simulink model "vertical_smm_3d_with_xz_lqr"  (R2015a)
settings: Solver=FixedStepDiscrete  SolverMode=SingleTasking  StartTime=0.0  StopTime=inf  FixedStep=sample_time  RelTol=1e-3
values from neighbouring files (symbols this model uses):
  forward_dx_of_dxstar = [-1.33773437568 -1.28773437515 -1.23773437461 -1.18773437408 -1.13773437355 -1.08773437301 -1.03773437248 -0.987734371946 -0.937734371413 -0.887734370879 -0.837734370532 -0.787734370254 ... (27552 elements, 41x21x32)]    [ref_trajs.mat]
  forward_x_of_dxstar = [0.243075305346 0.235858801492 0.228642297639 0.221425793786 0.214209289933 0.206992786079 0.199776282226 0.192559778373 0.18534327452 0.178126770666 0.17091026684 0.163693763058 ... (27552 elements, 41x21x32)]    [ref_trajs.mat]
  target_dx_range = [-1 -0.95 -0.9 -0.85 -0.8 -0.75 -0.7 -0.65 -0.6 -0.55 -0.5 -0.45 ... (41 elements, 1x41)]    [ref_trajs.mat]
undefined symbols (not defined in the file or in its folder): A1_notch_f1, A2_notch_f1, A_kalman_fourbar_gear, A_kalman_swing_load, A_kalman_transverse, A_kalman_vertical, A_lpf_accelerometer, A_lpf_dtau, A_lpf_fourbar_angles, A_lpf_imu, A_lpf_lateral_angle, B1_lpf_accelerometer, B1_lpf_dtau, B1_lpf_fourbar_angles, B1_lpf_imu, B1_lpf_lateral_angle, B1_notch_f1, B2_lpf_accelerometer, B2_lpf_dtau, B2_lpf_fourbar_angles, B2_lpf_imu, B2_lpf_lateral_angle, B2_notch_f1, B_dx_versus_x0, B_kalman_fourbar_gear, B_kalman_swing_load, B_kalman_transverse, B_kalman_vertical, backwards_K_sag_of_t, backwards_P_sag_of_t, C_kalman_fourbar_gear, C_kalman_swing_load, C_kalman_transverse, C_kalman_vertical, com_leg_motor, com_torso, contact_threshold, control_start_time, d_ankle_to_foot, d_vertical_com, desired_com_forward_velocity, desired_com_lateral_velocity, desired_initial_leg_roll_left, desired_initial_leg_roll_right, desired_stance_beta2, desired_standing_torso_pitch, desired_standing_torso_roll, desired_standing_z, desired_torso_pitch, desired_torso_roll, Discrete, enable_bouncing, fcut_contact, fdesignblkfcn, g, gcbh, HIP_MTR_MAX_CONT_TORQUE, HIP_MTR_MAX_TORQUE, i_leg_motor, i_robot ... (+91)
libraries: simulink x33, ctrlSharedLib x11, dsparch4 x10, dspfdesign x2
(part 1 of 7)
settings Model: CovSFcnEnable=off  Creator=wmartin  LastModifiedBy=wmartin
settings SolverCC: EnableConcurrentExecution=on
settings DataIOCC: LimitDataPoints=off  MaxDataPoints=1000000000  SaveFormat=StructureWithTime  SignalLogging=off  DSMLogging=off  VisualizeSimOutput=off
settings OptimizationCC: BlockReduction=off  OptimizeBlockIOStorage=off  BufferReuse=off  GlobalBufferReuse=off  ExpressionFolding=off  ExpressionDepthLimit=2147483647  LocalBlockOutputs=off  SimCompilerOptimization=on
settings DebuggingCC: UnderspecifiedInitializationDetection=Classic  MergeDetectMultiDrivingBlocksExec=none  SolverPrmCheckMsg=warning  StateNameClashWarn=warning
settings HardwareCC: ProdIntDivRoundTo=Zero  ProdEndianess=LittleEndian  ProdLongLongMode=on  ProdHWDeviceType=Generic->32-bit x86 compatible
settings ModelReferenceCC: UpdateModelReferenceTargets=IfOutOfDate  ModelReferenceNumInstancesAllowed=Single  ModelReferenceMinAlgLoopOccurrences=on
settings RTWCC: SystemTargetFile=slrt.tlc  TemplateMakefile=slrt_default_tmf  Description=Simulink Real-Time  RTWVerbose=off  RTWCompilerOptimization=on
settings CodeAppCC: MaxIdLength=256
settings SimulinkRealTimeCC: GeneratePreprocessorConditionals=Disable all  RL32LogBufSizeModifier=1e8

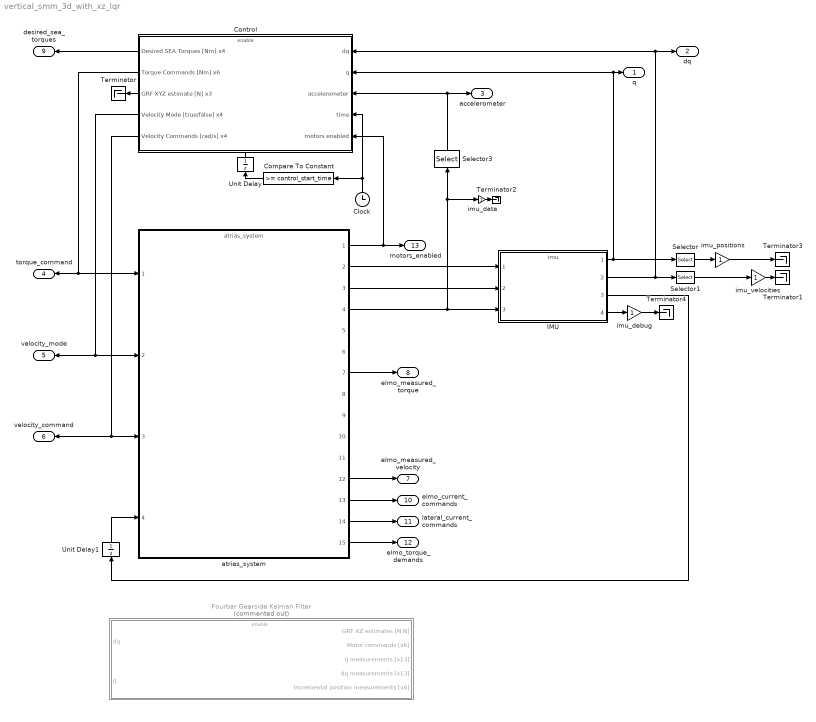
== system vertical_smm_3d_with_xz_lqr ==
  Clock : Clock
  Compare To Constant : simulink/Logic and Bit Operations/Compare To Constant  relop=>=  const=control_start_time  OutDataTypeStr=boolean
  Control : Subsystem
  Fourbar Gearside Kalman Filter : Subsystem  Commented=on
  IMU : ModelReference  ModelNameDialog=imu  SimulationMode=Normal  ModelReferenceVersion=1.2455  CopyOfModelName=imu  DefaultDataLogging=on
  Selector : Selector  InputPortWidth=13  Indices=[11 12 13]
  Selector1 : Selector  InputPortWidth=13  Indices=[11 12 13]
  Selector3 : Selector  InputPortWidth=9  Indices=[4 5 6]
  Terminator{,1..4} (5 alike) : Terminator
  Unit Delay : UnitDelay  SampleTime=-1
  Unit Delay1 : UnitDelay  SampleTime=-1
  atrias_system : ModelReference  ModelNameDialog=atrias_system  SimulationMode=Normal  ModelReferenceVersion=1.2965  CopyOfModelName=atrias_system  DefaultDataLogging=on
  imu_data : Gain
  imu_debug : Gain
  imu_positions : Gain
  imu_velocities : Gain
  q : Outport  SampleTime=sample_time
  dq : Outport  Port=2  SampleTime=sample_time
  accelerometer : Outport  Port=3  SampleTime=sample_time
  torque_command : Outport  Port=4  SampleTime=sample_time
  velocity_mode : Outport  Port=5  SampleTime=sample_time
  velocity_command : Outport  Port=6  SampleTime=sample_time
  elmo_measured_velocity : Outport  Port=7  SampleTime=sample_time
  elmo_measured_torque : Outport  Port=8  SampleTime=sample_time
  desired_sea_torques : Outport  Port=9  SampleTime=sample_time
  elmo_current_commands : Outport  Port=10  SampleTime=sample_time
  lateral_current_commands : Outport  Port=11  SampleTime=sample_time
  elmo_torque_demands : Outport  Port=12  SampleTime=sample_time
  motors_enabled : Outport  Port=13  SampleTime=sample_time
  wires:
  Compare To Constant/1 -> Unit Delay/1
  imu_data/1 -> Terminator2/1
  imu_velocities/1 -> Terminator1/1
  imu_positions/1 -> Terminator3/1
  imu_debug/1 -> Terminator4/1
  IMU/4 -> imu_debug/1
  Selector/1 -> imu_positions/1
  Selector1/1 -> imu_velocities/1
  atrias_system/2 -> IMU/1
  IMU/1 -> Selector/1, Control/2(q), q/1
  Control/2(Torque Commands [Nm] x6) -> atrias_system/1, torque_command/1
  atrias_system/3 -> IMU/2
  atrias_system/4 -> Selector3/1, imu_data/1, IMU/3
  IMU/3 -> Unit Delay1/1
  Unit Delay/1 -> Control/Enable
  IMU/2 -> Selector1/1, Control/1(dq), dq/1
  Control/5(Velocity Commands [rad/s] x4) -> velocity_command/1, atrias_system/3
  Control/4(Velocity Mode [true/false] x4) -> velocity_mode/1, atrias_system/2
  Selector3/1 -> Control/3(accelerometer), accelerometer/1
  Control/1(Desired SEA Torques [Nm] x4) -> desired_sea_torques/1
  Clock/1 -> Control/4(time), Compare To Constant/1
  Control/3(GRF XYZ estimate [N] x3) -> Terminator/1
  atrias_system/15 -> elmo_torque_demands/1
  atrias_system/14 -> lateral_current_commands/1
  atrias_system/13 -> elmo_current_commands/1
  atrias_system/12 -> elmo_measured_velocity/1
  atrias_system/7 -> elmo_measured_torque/1
  atrias_system/1 -> Control/5(motors enabled), motors_enabled/1
  Unit Delay1/1 -> atrias_system/4

== system vertical_smm_3d_with_xz_lqr/Control ==
  dq : Inport
  q : Inport  Port=2
  accelerometer : Inport  Port=3
  time : Inport  Port=4
  motors enabled : Inport  Port=5
  Enable : EnablePort  StatesWhenEnabling=reset  PropagateVarSize=During execution  ShowOutputPort=on
  Actuator Control : ModelReference  ModelNameDialog=actuator_control  SimulationMode=Normal  ModelReferenceVersion=1.1249  CopyOfModelName=actuator_control  DefaultDataLogging=on
  Actuator Control with Torque SEA commands : Subsystem  Commented=on
  Behavior Control : Subsystem
  Compute Body Frame Accelerations : Subsystem
  Detect Change : simulink/Logic and Bit Operations/Detect Change  vinit=0  InputProcessing=Inherited  OutDataTypeStr=boolean
  Filter Velocities : Subsystem
  Mux : Mux
  Desired SEA Torques [Nm] x4 : Outport  InitialOutput=[0 0 0 0]
  Torque Commands [Nm] x6 : Outport  Port=2  InitialOutput=[0 0 0 0 0 0]
  GRF XYZ estimate [N] x3 : Outport  Port=3  InitialOutput=[0 0 0]
  Velocity Mode [true/false] x4 : Outport  Port=4  InitialOutput=[false false false false]
  Velocity Commands [rad/s] x4 : Outport  Port=5  InitialOutput=[0 0 0 0]
  wires:
  Behavior Control/1(Torque Commands [Nm] x6) -> Actuator Control/2
  Behavior Control/2(Velocity Commands [rad/s] x4) -> Actuator Control/3
  Behavior Control/3(Stance / Swing Control [1/0] x4) -> Actuator Control/4
  time/1 -> Actuator Control/5, Behavior Control/5(time)
  Detect Change/1 -> Mux/1, Mux/2, Mux/3, Mux/4
  motors enabled/1 -> Detect Change/1
  Mux/1 -> Actuator Control/1
  Actuator Control/4 -> Desired SEA Torques [Nm] x4/1
  Enable/1 -> Behavior Control/1(Enabled [true/false])
  Compute Body Frame Accelerations/1(accelerations [m/s^2] x3) -> Behavior Control/2(Body XYZ Acceleration [m/s^2] x3)
  accelerometer/1 -> Compute Body Frame Accelerations/1(accelerometer [g] x3)
  Actuator Control/3 -> Velocity Commands [rad/s] x4/1
  Actuator Control/2 -> Velocity Mode [true/false] x4/1
  dq/1 -> Actuator Control/7, Filter Velocities/1(raw dq)
  Filter Velocities/1(filtered dq) -> Behavior Control/3(dq)
  Behavior Control/4(GRF XYZ estimates [N N N]) -> GRF XYZ estimate [N] x3/1
  Actuator Control/1 -> Torque Commands [Nm] x6/1
  q/1 -> Actuator Control/6, Behavior Control/4(q)

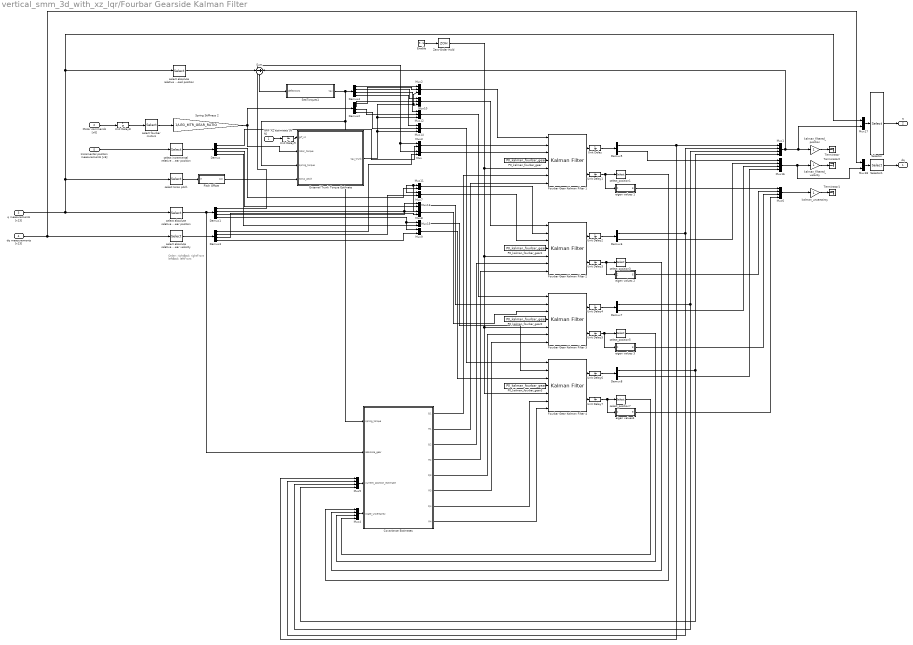
== system vertical_smm_3d_with_xz_lqr/Fourbar Gearside Kalman Filter ==
  note: Order:
      | rightBack
      | rightFront
      | leftBack
      | leftFront
  GRF XZ estimates [N N] : Inport  SampleTime=sample_time
  Motor commands [x6] : Inport  Port=2  SampleTime=sample_time
  q measurements [x13] : Inport  Port=3  SampleTime=sample_time
  dq measurements [x13] : Inport  Port=4  SampleTime=sample_time
  Incremental position measurements [x6] : Inport  Port=5  SampleTime=sample_time
  Enable : EnablePort  ShowOutputPort=on
  Covariance Estimates : MATLAB Function  TreatAsAtomicUnit=on
  Demux{,1..4} (5 alike) : Demux
  Demux{5..8} (4 alike) : Demux  Outputs=2
  External Trunk Torque Estimate : MATLAB Function  TreatAsAtomicUnit=on
  Fourbar Gear Kalman Filter {1..4} (4 alike) : ctrlSharedLib/Kalman Filter  TimeDomain=Discrete-Time  UseCurrentEstimator=on  ModelSource=Individual A, B, C, D matrices  ModelSourceVariable=A_kf  A=A_kalman_fourbar_gear  B=B_kalman_fourbar_gear  C=C_kalman_fourbar_gear  D=0  NumberOfStates=2  NumberOfInputs=1  NumberOfOutputs=2  InitialEstimateSource=Input port  X0=initial_dx_estimate  P0=P0_kalman_transverse  UseK=off  UseGH=on  NumberOfProcessNoiseInputs=1  G=G_kalman_fourbar_gear  TimeInvariantG=on  H=0  TimeInvariantH=on  Q=1  TimeInvariantQ=off  R=1  TimeInvariantR=off  N=0  TimeInvariantN=on  AddInputPort=on  AddEnablePort=off  ExternalReset=Either  OutputEstimatedY=off  OutputP=on  Ts=sample_time
  Mux{,3,7..9,11,13,15,17..18} (10 alike) : Mux  Inputs=2
  Mux{1,4..6,16} (5 alike) : Mux
  Mux{2,10,12,14} (4 alike) : Mux  Inputs=3
  P0_kalman_fourbar_gear{,1..3} (4 alike) : Constant  Value=P0_kalman_fourbar_gear
  Pitch Offset : Subsystem
  SeaTorques1 : MATLAB Function  TreatAsAtomicUnit=on
  Selector : Selector  InputPortWidth=17  Indices=[1 14 3 15 5 16 7 17 9 10 11 12 13]
  Selector1 : Selector  InputPortWidth=17  Indices=[1 14 3 15 5 16 7 17 9 10 11 12 13]
  Spring Stiffness 2 : Gain  Gain=1/LEG_MTR_GEAR_RATIO
  Sum : Sum  Inputs=-|+
  Terminator : Terminator
  Terminator1 : Terminator
  Terminator2 : Terminator
  Unit Delay{,1..9} (10 alike) : UnitDelay  SampleTime=-1
  Zero-Order Hold : ZeroOrderHold  SampleTime=sample_time
  eigen values 1 : MATLAB Function  TreatAsAtomicUnit=on
  eigen values 2 : MATLAB Function  TreatAsAtomicUnit=on
  eigen values 3 : MATLAB Function  TreatAsAtomicUnit=on
  "eigen values4 " : MATLAB Function  TreatAsAtomicUnit=on
  kalman_filtered_position : Gain
  kalman_filtered_velocity : Gain
  kalman_uncertainty : Gain
  select absolute relative gear position : Selector  InputPortWidth=13  Indices=[2 4 6 8]
  select absolute relative gear velocity : Selector  InputPortWidth=13  Indices=[2 4 6 8]
  select absolute relative load position : Selector  InputPortWidth=13  Indices=[2 4 6 8]
  select fourbar motors : Selector  InputPortWidth=6  Indices=[1 2 3 4]
  select incremental relative gear position : Selector  InputPortWidth=6  Indices=[1 2 3 4]
  select torso pitch : Selector  InputPortWidth=13  Indices=[13]
  select_position{1,3,5,7} (4 alike) : Selector  NumberOfDimensions=2  InputPortWidth=2  IndexOptions=Index vector (dialog),Index vector (dialog)  Indices=[1],[1]  OutputSizes=1,1
  dq : Outport
  q : Outport  Port=2
  wires:
  select incremental relative gear position/1 -> Demux/1
  q measurements [x13]/1 -> select absolute relative gear position/1, Mux17/1, select absolute relative load position/1, select torso pitch/1
  Incremental position measurements [x6]/1 -> select incremental relative gear position/1
  Motor commands [x6]/1 -> Unit Delay8/1
  select fourbar motors/1 -> Spring Stiffness 2/1
  P0_kalman_fourbar_gear/1 -> Fourbar Gear Kalman Filter 1/4
  Mux/1 -> Fourbar Gear Kalman Filter 1/3
  select absolute relative gear velocity/1 -> Demux3/1
  dq measurements [x13]/1 -> Mux18/1, select absolute relative gear velocity/1
  Demux3/1 -> Mux/2
  GRF XZ estimates [N N]/1 -> Unit Delay9/1
  SeaTorques1/1(tau) -> Demux4/1, External Trunk Torque Estimate/3(spring_torque), Covariance Estimates/1(spring_torque)
  Fourbar Gear Kalman Filter 1/1 -> Unit Delay/1
  Demux5/1 -> Mux1/1, Mux5/1
  Mux1/1 -> Sum/2, Mux17/2, kalman_filtered_position/1
  select absolute relative load position/1 -> Sum/1
  Sum/1 -> SeaTorques1/1(deflections)
  External Trunk Torque Estimate/1(tau_trunk) -> Mux2/3, Mux10/3, Mux12/3, Mux14/3
  Demux4/1 -> Mux2/1
  Demux2/1 -> Mux2/2
  Mux2/1 -> Fourbar Gear Kalman Filter 1/1
  Demux/1 -> Mux3/2
  Demux1/1 -> Mux3/1, Mux/1
  Mux3/1 -> Fourbar Gear Kalman Filter 1/2
  Fourbar Gear Kalman Filter 1/2 -> Unit Delay1/1
  Mux4/1 -> Covariance Estimates/4(state_uncertainty)
  select absolute relative gear position/1 -> Covariance Estimates/2(absolute_gear), Demux1/1
  Mux5/1 -> Covariance Estimates/3(current_position_estimate)
  Covariance Estimates/1(Q1) -> Fourbar Gear Kalman Filter 1/6
  Covariance Estimates/2(R1) -> Fourbar Gear Kalman Filter 1/7
  select torso pitch/1 -> Pitch Offset/1(in)
  select_position1/1 -> Mux4/1
  P0_kalman_fourbar_gear1/1 -> Fourbar Gear Kalman Filter 2/4
  Fourbar Gear Kalman Filter 2/1 -> Unit Delay2/1
  Fourbar Gear Kalman Filter 2/2 -> Unit Delay3/1
  P0_kalman_fourbar_gear2/1 -> Fourbar Gear Kalman Filter 3/4
  Fourbar Gear Kalman Filter 3/1 -> Unit Delay4/1
  Fourbar Gear Kalman Filter 3/2 -> Unit Delay5/1
  P0_kalman_fourbar_gear3/1 -> Fourbar Gear Kalman Filter 4/4
  Fourbar Gear Kalman Filter 4/1 -> Unit Delay6/1
  Fourbar Gear Kalman Filter 4/2 -> Unit Delay7/1
  Covariance Estimates/3(Q2) -> Fourbar Gear Kalman Filter 2/6
  Covariance Estimates/5(Q3) -> Fourbar Gear Kalman Filter 3/6
  Covariance Estimates/7(Q4) -> Fourbar Gear Kalman Filter 4/6
  Covariance Estimates/4(R2) -> Fourbar Gear Kalman Filter 2/7
  Covariance Estimates/6(R3) -> Fourbar Gear Kalman Filter 3/7
  Covariance Estimates/8(R4) -> Fourbar Gear Kalman Filter 4/7
  select_position3/1 -> Mux4/2
  select_position5/1 -> Mux4/3
  select_position7/1 -> Mux4/4
  Demux6/1 -> Mux5/2, Mux1/2
  Demux7/1 -> Mux1/3, Mux5/3
  Demux8/1 -> Mux1/4, Mux5/4
  kalman_filtered_position/1 -> Terminator/1
  Enable/1 -> Zero-Order Hold/1
  Mux7/1 -> Fourbar Gear Kalman Filter 2/3
  Mux8/1 -> Fourbar Gear Kalman Filter 3/3
  Mux9/1 -> Fourbar Gear Kalman Filter 4/3
  Mux10/1 -> Fourbar Gear Kalman Filter 2/1
  Mux11/1 -> Fourbar Gear Kalman Filter 2/2
  Mux13/1 -> Fourbar Gear Kalman Filter 3/2
  Mux12/1 -> Fourbar Gear Kalman Filter 3/1
  Mux15/1 -> Fourbar Gear Kalman Filter 4/2
  Mux14/1 -> Fourbar Gear Kalman Filter 4/1
  Demux3/2 -> Mux7/2
  Demux3/3 -> Mux8/2
  Demux3/4 -> Mux9/2
  Demux1/2 -> Mux7/1, Mux11/1
  Demux1/3 -> Mux13/1, Mux8/1
  Demux1/4 -> Mux9/1, Mux15/1
  Demux/2 -> Mux11/2
  Demux/3 -> Mux13/2
  Demux/4 -> Mux15/2
  Demux4/2 -> Mux10/1
  Demux4/3 -> Mux12/1
  Demux4/4 -> Mux14/1
  Demux2/2 -> Mux10/2
  Demux2/3 -> Mux12/2
  Demux2/4 -> Mux14/2
  kalman_uncertainty/1 -> Terminator1/1
  Mux6/1 -> kalman_uncertainty/1
  kalman_filtered_velocity/1 -> Terminator2/1
  Mux16/1 -> Mux18/2, kalman_filtered_velocity/1
  Demux5/2 -> Mux16/1
  Demux6/2 -> Mux16/2
  Demux7/2 -> Mux16/3
  Demux8/2 -> Mux16/4
  Zero-Order Hold/1 -> Fourbar Gear Kalman Filter 4/5, Fourbar Gear Kalman Filter 3/5, Fourbar Gear Kalman Filter 2/5, Fourbar Gear Kalman Filter 1/5
  Unit Delay1/1 -> eigen values 1/1(Z), select_position1/1
  Unit Delay3/1 -> eigen values 2/1(Z), select_position3/1
  Unit Delay4/1 -> Demux7/1
  Unit Delay7/1 -> "eigen values4 "/1(Z), select_position7/1
  Unit Delay6/1 -> Demux8/1
  Spring Stiffness 2/1 -> Demux2/1, External Trunk Torque Estimate/2(rotor_torque)
  Unit Delay5/1 -> eigen values 3/1(Z), select_position5/1
  eigen values 1/1(E) -> Mux6/1
  eigen values 2/1(E) -> Mux6/2
  eigen values 3/1(E) -> Mux6/3
  "eigen values4 "/1(E) -> Mux6/4
  Unit Delay/1 -> Demux5/1
  Unit Delay2/1 -> Demux6/1
  Mux17/1 -> Selector/1
  Selector/1 -> q/1
  Selector1/1 -> dq/1
  Mux18/1 -> Selector1/1
  Unit Delay8/1 -> select fourbar motors/1
  Unit Delay9/1 -> External Trunk Torque Estimate/1(grf_xz)
  Pitch Offset/1(out) -> External Trunk Torque Estimate/4(torso_pitch)

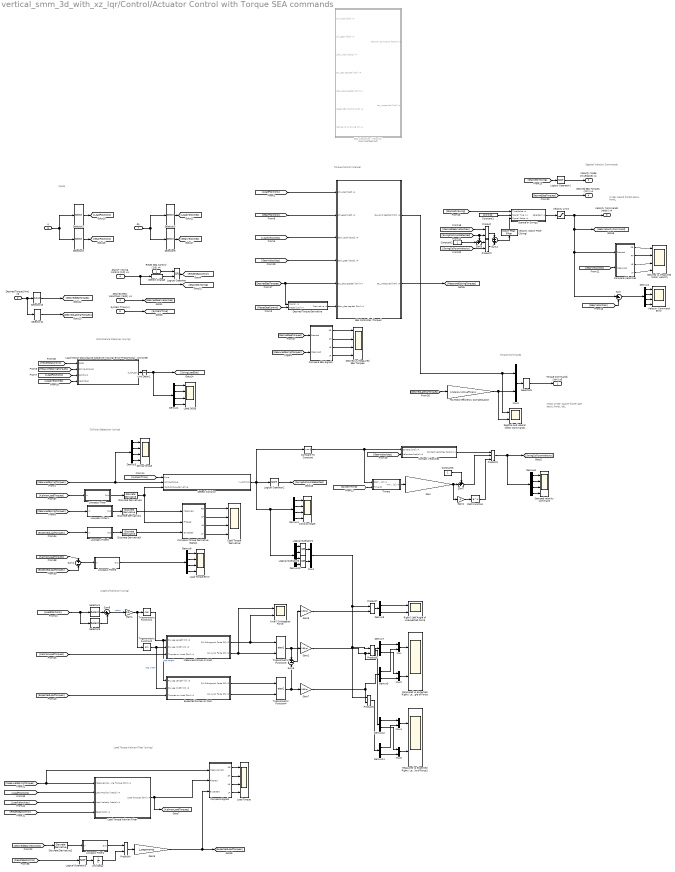
== system vertical_smm_3d_with_xz_lqr/Control/Actuator Control with Torque SEA commands ==
  note: Angle of Collision (swing)
  note: Load Torque Kalman Filter (swing)
  note: Collision Detection (swing)
  note: Sagittal Velocity Commands
  note: Torque Commands
  note: Disturbance Observer (swing)
  note: Inputs
  note: Torque Control (stance)
  note: Motor Order:
      |
      | backR
      | frontR
      | latR
      | backL
      | frontL
      | latL
  note: Order:
      | backR
      | frontR
      | backL
      | frontL
  Reset SEA Control [1/0] x4 : Inport  OutDataTypeStr=boolean  PortDimensions=4  SampleTime=sample_time
  Desired Torque [Nm] x6 : Inport  Port=2  OutDataTypeStr=double  PortDimensions=6  SampleTime=sample_time
  Desired Gear Velocities [rad/s] x4 : Inport  Port=3  OutDataTypeStr=double  PortDimensions=4  SampleTime=sample_time
  Stance / Swing Control [1/0] x4 : Inport  Port=4  OutDataTypeStr=boolean  PortDimensions=4  SampleTime=sample_time
  System Time [s] : Inport  Port=5  OutDataTypeStr=double  PortDimensions=1  SampleTime=sample_time
  q : Inport  Port=6  OutDataTypeStr=double  PortDimensions=13  SampleTime=sample_time
  dq : Inport  Port=7  OutDataTypeStr=double  PortDimensions=13  SampleTime=sample_time
  Axial / Orthogonal Force : Scope  NumInputPorts=2
      settings: YMin=-120~-175  YMax=120~150  SampleInput=on
  Collision State : Scope  NumInputPorts=4
      settings: YMin=0~-4~-1~-2.25  YMax=6~4~0.75~0  SaveName=LoadDOB_history2  SampleInput=on
  Compare To Constant : simulink/Logic and Bit Operations/Compare To Constant  relop=~=  const=0  OutDataTypeStr=boolean
  Compare SEA Signals : Subsystem
  Compare Signals : Subsystem
  Compare Torque Derivative Signals : Subsystem
  Compare Velocities : Subsystem
  Constant1 : Constant  Value=[0 0 0 0]
  Constant2 : Constant
  Constant5 : Constant
  Contact Velocities : Subsystem
  Damped velocity command : Scope  NumInputPorts=4
      settings: YMin=0~-4~-1~-2.25  YMax=6~4~0.75~0  SaveName=LoadDOB_history6  SampleInput=on
  Demux{1..4,6,8,10} (7 alike) : Demux
  Demux{5,7,9,11..12} (5 alike) : Demux  Outputs=2
  Desired Torque Derivative : Subsystem
  Desired vs Measured Motor Velocity : Scope  NumInputPorts=4
      settings: YMin=-0.03~-0.03~-0.025~-0.025  YMax=0.02~0.025~0.02~0.02  SaveName=ScopeData14  SampleInput=on
  Desired vs Measured SEA Torques : Scope  NumInputPorts=4
      settings: YMin=-35~-75~-500~-200  YMax=50~75~150~550  SaveName=SeaTorques  SampleInput=on  SampleTime=sample_time
  Detect Change : simulink/Logic and Bit Operations/Detect Change  vinit=0  InputProcessing=Inherited  OutDataTypeStr=boolean
  Detect Collision : MATLAB Function  TreatAsAtomicUnit=on
  Discrete Derivative{1..4} (4 alike) : simulink/Discrete/Discrete Derivative  gainval=1.0  ICPrevScaledInput=0.0  OutMin=[]  OutMax=[]  OutDataType=fixdt(1, 16)  OutScaling=2^-10  DoSatur=off
  Expected Forces on Foot : Subsystem
  Gain : Gain  Gain=swing_collision_damping_rate
  Gain1 : Gain  Gain=-1
  Gain2 : Gain  Gain=180/pi
  Gain4 : Gain  Gain=0.5
  Gain5 : Gain  Gain=j_segments
  Gain6 : Gain  Gain=180/pi
  Gain7 : Gain  Gain=180/pi
  Hip Motor Efficiency Compensation : Gain  Gain=1/lateral_motor_efficiency
  Load DOBs : Scope  NumInputPorts=4
      settings: YMin=-12~-7~2.7~-0.5  YMax=-8.75~1~4.1~2  SaveName=LoadDOB_history  SampleInput=on
  Load Motion Disturbance Observer (Swing) Error-Proportional - 2nd order : MATLAB Function  TreatAsAtomicUnit=on
  Load Torque : Scope  NumInputPorts=4
      settings: TimeRange=34.366  YMin=-300~-400~-100~-200  YMax=100~150~400~800  SaveName=LoadDOB_history3  SampleInput=on
  Load Torque Derivative : Scope  NumInputPorts=4
      settings: TimeRange=50.096  YMin=-4122.660296851378~-4185.660018993349~-3974.358974358969~-4680.851063829847  YMax=3871.203105284947~4522.792022792026~4743.58974358975~5531.914893616988  SaveName=LoadDOB_history4  SampleInput=on
  Load Torque Error : Scope  NumInputPorts=4
      settings: YMin=-100~-125~-125~-125  YMax=125~100~125~100  SaveName=LoadDOB_history5  SampleInput=on
  Load Torque Kalman Filter : Subsystem
  Logical Operator : Logic  Operator=OR  AllPortsSameDT=off  OutDataTypeStr=boolean
  Logical Operator1 : Logic  Operator=NOT  AllPortsSameDT=off  OutDataTypeStr=boolean
  Logical Operator2 : Logic  Operator=NOT  AllPortsSameDT=off  OutDataTypeStr=boolean
  Logical Operator3 : Logic  Operator=NOT  AllPortsSameDT=off  OutDataTypeStr=boolean
  Logical Operator4 : Logic  Operator=OR  AllPortsSameDT=off  OutDataTypeStr=boolean
  Logical Operator5 : Logic  Operator=OR  AllPortsSameDT=off  OutDataTypeStr=boolean
  Lowpass Filter : Subsystem  DialogController=fdesignblkfcn  InitFcn=fdesignblkfcn(gcbh, {'InitFcn'});  mask(Lowpass Filter){}
      mask help: Design a lowpass filter
      settings: CopyFcn=fdesignblkfcn(gcbh, {'CopyFcn'});
      mask Help: helpview(mapfilelocation('dsp'), 'dsplowpassfilter');
      mask Display: disp('Lowpass')
  Lowpass Filter1 : Subsystem  DialogController=fdesignblkfcn  InitFcn=fdesignblkfcn(gcbh, {'InitFcn'});  mask(Lowpass Filter){}
      mask help: Design a lowpass filter
      settings: CopyFcn=fdesignblkfcn(gcbh, {'CopyFcn'});
      mask Help: helpview(mapfilelocation('dsp'), 'dsplowpassfilter');
      mask Display: disp('Lowpass')
  Lowpass Filter2 : Subsystem  DialogController=fdesignblkfcn  InitFcn=fdesignblkfcn(gcbh, {'InitFcn'});  mask(Lowpass Filter){}
      mask help: Design a lowpass filter
      settings: CopyFcn=fdesignblkfcn(gcbh, {'CopyFcn'});
      mask Help: helpview(mapfilelocation('dsp'), 'dsplowpassfilter');
      mask Display: disp('Lowpass')
  Lowpass Filter5 : Subsystem  DialogController=fdesignblkfcn  InitFcn=fdesignblkfcn(gcbh, {'InitFcn'});  mask(Lowpass Filter){}
      mask help: Design a lowpass filter
      settings: CopyFcn=fdesignblkfcn(gcbh, {'CopyFcn'});
      mask Help: helpview(mapfilelocation('dsp'), 'dsplowpassfilter');
      mask Display: disp('Lowpass')
  Lowpass Filter6 : Subsystem  DialogController=fdesignblkfcn  InitFcn=fdesignblkfcn(gcbh, {'InitFcn'});  mask(Lowpass Filter){}
      mask help: Design a lowpass filter
      settings: CopyFcn=fdesignblkfcn(gcbh, {'CopyFcn'});
      mask Help: helpview(mapfilelocation('dsp'), 'dsplowpassfilter');
      mask Display: disp('Lowpass')
  Math Function : Math  SaturateOnIntegerOverflow=on
  Measured Forces on Foot : Subsystem
  Measured vs Expected Right / Left Angle of Force : Scope  NumInputPorts=2
      settings: TimeRange=45  YMin=-200~-200  YMax=200~200  SampleInput=on
  Measured vs Expected Right / Left Angle of Force1 : Scope  NumInputPorts=2
      settings: TimeRange=45  YMin=-1~-200  YMax=1~200  SaveName=ScopeData8  SampleInput=on
  Mux{,1..5} (6 alike) : Mux  Inputs=2
  Product{,2,4..7} (6 alike) : Product
  Product3 : Product  Inputs=3
  Right / Left Angle of Unexpected Force : Scope  NumInputPorts=2
      settings: TimeRange=45  YMin=-350~-400  YMax=300~350  SaveName=ScopeData3  SampleInput=on
  SEA Controller (Torque) : Subsystem
  SEA Controller (Velocity) : Subsystem  Commented=on
  Sagittal and Lateral Motor Commands : Scope  NumInputPorts=2
      settings: YMin=-1~0  YMax=1~65  SaveName=ScopeData2  SampleInput=on
  Selector1 : Selector  InputPortWidth=13  Indices=[1 3 5 7]
  Selector10 : Selector  InputPortWidth=6  Indices=[1 2 4 5]
  Selector11 : Selector  InputPortWidth=6  Indices=[3 6]
  Selector3 : Selector  InputPortWidth=13  Indices=[2 4 6 8]
  Selector4 : Selector  InputPortWidth=4  Indices=[1 3]
  Selector5 : Selector  InputPortWidth=13  Indices=[1 3 5 7]
  Selector6 : Selector  InputPortWidth=4  Indices=[2 4]
  Selector8 : Selector  InputPortWidth=6  Indices=[1 2 5 3 4 6]
  Selector9 : Selector  InputPortWidth=13  Indices=[2 4 6 8]
  Spring Torque : Scope  NumInputPorts=4
      settings: YMin=-75~-75~-75~-75  YMax=75~75~75~75  SaveName=LoadDOB_history1  SampleInput=on
  Stance or Swing1 : Subsystem
  Sum : Sum  Inputs=|+-
  Sum2 : Sum  Inputs=+|-
  Sum3 : Sum  Inputs=-+|
  Sum4 : Sum  Inputs=+|+
  Sum6 : Sum  Inputs=+|-
  Sum7 : Sum  Inputs=++|
  Sum8 : Sum  Inputs=|+-
  Timers : Subsystem
  Trigonometric Function1 : Trigonometry  Operator=cos
  Trigonometric Function2 : Trigonometry
  Trigonometric Function3 : Trigonometry  Operator=atan2
  Trigonometric Function4 : Trigonometry  Operator=atan2
  Unit Delay : UnitDelay  SampleTime=-1
  Unit Delay1 : UnitDelay  SampleTime=sample_time
  Velocity Command Error : Scope  NumInputPorts=4
      settings: YMin=-0.5~-0.4~-0.5~-1.5  YMax=1.5~0.5~0.9~0.75  SaveName=ScopeData6  SampleInput=on
  Velocity Limit : Saturate  UpperLimit=8  LowerLimit=-8
      settings: AttributesFormatString=Hi: %<UpperLimit>\nLo: %<LowerLimit>
  Velocity Notch Filter (Swing) : dspfdesign/Notch-Peak Filter  Specification=Quality factor and center frequency  Bandwidth=27  QualityFactor=2.5  CenterFrequency=27  BandwidthCoefficient=0.72654  CenterFrequencyCoefficient=0  Output=Notch  InheritSampleRate=off  SampleRate=update_freq  SimulateUsing=Code generation
  Torque Commands [Nm] x6 : Outport  OutDataTypeStr=double  PortDimensions=6  SampleTime=0  InitialOutput=[0 0 0 0 0 0]
  Velocity Mode [true/false] x4 : Outport  Port=2  InitialOutput=[false false false false]
  Velocity Commands [rad/s] x4 : Outport  Port=3  InitialOutput=[0 0 0 0]
  Desired SEA Torques [Nm] x4 : Outport  Port=4  InitialOutput=[false false false false]
  wires:
  [MeasuredSpringTorques] -> Detect Collision/2(spring_torque), Demux3/1
  Velocity Limit/1 -> Compare Velocities/1(Desired), Sum/1, [GearVelocityCommand], Velocity Commands [rad/s] x4/1
  Velocity Notch Filter (Swing)/1 -> Stance or Swing1/3(Signal False x4)
  Product5/1 -> Demux11/1
  Product6/1 -> Demux12/1
  Mux4/1 -> Measured vs Expected Right / Left Angle of Force1/1
  Mux5/1 -> Measured vs Expected Right / Left Angle of Force1/2
  Demux11/1 -> Mux4/2
  Demux11/2 -> Mux5/2
  Demux12/1 -> Mux4/1
  Demux12/2 -> Mux5/1
  Product7/1 -> Demux9/1
  Sum6/1 -> Gain6/1
  Mux1/1 -> Product6/1, Product5/1, Product7/1
  Gain2/1 -> Product6/2, Demux7/1
  Gain7/1 -> Product5/2, Demux5/1
  Mux/1 -> Measured vs Expected Right / Left Angle of Force/1
  Mux2/1 -> Measured vs Expected Right / Left Angle of Force/2
  Expected Forces on Foot/2(R/L Axial Force [N] x2) -> Trigonometric Function4/2
  Demux9/2 -> Right / Left Angle of Unexpected Force/2
  Demux9/1 -> Right / Left Angle of Unexpected Force/1
  Gain6/1 -> Product7/2
  Trigonometric Function4/1 -> Gain7/1, Sum6/2
  Expected Forces on Foot/1(R/L Orthogonal Force [N] x2) -> Trigonometric Function4/1
  [ExpectedLoadTorques] -> Expected Forces on Foot/3(Torques on Load [Nm] x4)
  Measured Forces on Foot/2(R/L Axial Force [N] x2) -> Trigonometric Function3/2, Axial / Orthogonal Force/1
  Measured Forces on Foot/1(R/L Orthogonal Force [N] x2) -> Axial / Orthogonal Force/2, Trigonometric Function3/1
  [KalmanLoadTorques] -> Measured Forces on Foot/3(Torques on Load [Nm] x4)
  Trigonometric Function2/1 -> Expected Forces on Foot/2(R/L Leg Width [m] x2), Measured Forces on Foot/2(R/L Leg Width [m] x2)  "leg width"
  Trigonometric Function1/1 -> Measured Forces on Foot/1(R/L Leg Length [m] x2), Expected Forces on Foot/1(R/L Leg Length [m] x2)  "leg length"
  Lowpass Filter2/1(Out) -> Product4/1
  Lowpass Filter/1(Out) -> Discrete Derivative1/1
  Lowpass Filter6/1(Out) -> Demux6/1
  Discrete Derivative1/1 -> Detect Collision/3(load_torque_derivative), Compare Torque Derivative Signals/2(Filtered)
  Sum7/1 -> Product3/2
  Logical Operator5/1 -> Mux1/2
  Logical Operator4/1 -> Mux1/1
  Demux10/3 -> Logical Operator5/1
  Demux10/4 -> Logical Operator5/2
  Demux10/2 -> Logical Operator4/2
  Demux10/1 -> Logical Operator4/1
  Demux5/1 -> Mux/2
  Demux5/2 -> Mux2/2
  Selector6/1 -> Sum8/2
  Discrete Derivative3/1 -> Compare Torque Derivative Signals/3(Expected)
  [DesiredGearVelocities] -> Discrete Derivative2/1
  Sum2/1 -> Lowpass Filter6/1(In)
  [ExpectedLoadTorques] -> Sum2/2
  [KalmanLoadTorques] -> Sum2/1
  Demux6/4 -> Load Torque Error/4
  Demux6/1 -> Load Torque Error/1
  Demux6/2 -> Load Torque Error/2
  Demux6/3 -> Load Torque Error/3
  Discrete Derivative4/1 -> Compare Torque Derivative Signals/1(Measured)
  Lowpass Filter1/1(Out) -> Discrete Derivative4/1
  [MeasuredSpringTorques] -> Lowpass Filter1/1(In)
  Compare Torque Derivative Signals/1(RB) -> Load Torque Derivative/1
  Compare Torque Derivative Signals/2(RF) -> Load Torque Derivative/2
  Compare Torque Derivative Signals/3(LB) -> Load Torque Derivative/3
  Compare Torque Derivative Signals/4(LF) -> Load Torque Derivative/4
  Lowpass Filter5/1(Out) -> Discrete Derivative3/1
  [ExpectedLoadTorques] -> Lowpass Filter5/1(In)
  Unit Delay/1 -> Product4/2
  [ResetSeaControl] -> Logical Operator3/1
  Logical Operator3/1 -> Unit Delay/1
  Discrete Derivative2/1 -> Lowpass Filter2/1(In)
  Gain5/1 -> Compare Signals/3(Expected), [ExpectedLoadTorques]
  Product4/1 -> Gain5/1
  Trigonometric Function3/1 -> Gain2/1, Sum6/1
  [LoadPositions] -> Load Torque Kalman Filter/2(Load Position [rad/s] x4)
  [MeasuredSpringTorques] -> Load Torque Kalman Filter/1(Measured Spring Torque [Nm] x4), Compare Signals/1(Measurement)
  Load Torque Kalman Filter/1(Load Torques [Nm] x4) -> Compare Signals/2(Filtered), [KalmanLoadTorques]
  Compare Signals/1(RB) -> Load Torque/1
  Compare Signals/4(LF) -> Load Torque/4
  Compare Signals/2(RF) -> Load Torque/2
  Compare Signals/3(LB) -> Load Torque/3
  [ResetSeaControl] -> Load Torque Kalman Filter/4(Reset [1/0] x4)
  [LoadVelocities] -> Load Torque Kalman Filter/3(Load Velocity [rad/s] x4)
  Demux7/1 -> Mux/1
  Demux7/2 -> Mux2/1
  [LoadPositions] -> Selector4/1, Selector6/1
  Gain4/1 -> Trigonometric Function1/1, Trigonometric Function2/1
  Sum8/1 -> Gain4/1  "splay"
  Selector4/1 -> Sum8/1
  Logical Operator2/1 -> [SwingCollisionDetected]
  Demux4/4 -> Collision State/4
  Demux4/1 -> Collision State/1
  Demux4/2 -> Collision State/2
  Demux4/3 -> Collision State/3
  [SystemTime] -> Detect Collision/1(time)
  System Time [s]/1 -> [SystemTime]
  Selector9/1 -> [GearVelocities]
  Sum4/1 -> Velocity Notch Filter (Swing)/1
  [SystemTime] -> Timers/2(Time [s])
  Demux8/4 -> Damped velocity command/4
  Demux8/1 -> Damped velocity command/1
  Demux8/2 -> Damped velocity command/2
  Demux8/3 -> Damped velocity command/3
  Product3/1 -> Demux8/1, [SwingCollisionVelocity]
  Math Function/1 -> Product3/3
  Gain1/1 -> Math Function/1
  Constant5/1 -> Sum7/1
  Gain/1 -> Sum7/2, Gain1/1
  Timers/1(Timer [s] x4) -> Gain/1
  Compare To Constant/1 -> Timers/1(Start [1/0] x4), Contact Velocities/1(Contact [1/0] x4)
  Contact Velocities/1(Contact Velocities [rad/s] x4) -> Product3/1
  [GearVelocities] -> Contact Velocities/2(Velocities [rad/s] x4)
  Desired Gear Velocities [rad/s] x4/1 -> [DesiredGearVelocities]
  Detect Change/1 -> Logical Operator/2
  [StanceOrSwing] -> Stance or Swing1/1(True/False x4)
  Stance or Swing1/1(Selected x4) -> Velocity Limit/1
  Detect Collision/1(in_collision) -> Logical Operator2/1, Demux4/1, Demux10/1, Compare To Constant/1
  [KalmanLoadTorques] -> Lowpass Filter/1(In)
  Sum3/1 -> Product2/1
  Product2/1 -> Sum4/2
  Product/1 -> Sum4/1
  [SwingCollisionVelocity] -> Product2/2
  Constant2/1 -> Sum3/2
  Selector10/1 -> [DesiredSeaTorques]
  [SwingCollisionDetected] -> Product/2, Sum3/1
  Demux3/1 -> Spring Torque/1
  Demux3/2 -> Spring Torque/2
  Demux3/3 -> Spring Torque/3
  Demux3/4 -> Spring Torque/4
  Demux2/1 -> Velocity Command Error/1
  Demux2/2 -> Velocity Command Error/2
  Demux2/3 -> Velocity Command Error/3
  Demux2/4 -> Velocity Command Error/4
  [DesiredGearVelocities] -> Product/1
  Sum/1 -> Demux2/1
  [GearVelocities] -> Sum/2
  [GearVelocities] -> Compare Velocities/2(Measured)
  [GearPositions] -> SEA Controller (Torque)/2(phi_gear [rad] x4)
  dq/1 -> Selector9/1, Selector5/1
  Selector3/1 -> [GearPositions]
  [LoadVelocities] -> SEA Controller (Torque)/3(dphi_load [rad/s] x4)
  [DesiredSeaTorques] -> Desired SEA Torques [Nm] x4/1
  Reset SEA Control [1/0] x4/1 -> Logical Operator/1
  Logical Operator/1 -> [ResetSeaControl]
  Stance / Swing Control [1/0] x4/1 -> Detect Change/1, [StanceOrSwing]
  Unit Delay1/1 -> Demux1/1, [SwingLoadDob]
  Demux1/4 -> Load DOBs/4
  Demux1/3 -> Load DOBs/3
  Demux1/2 -> Load DOBs/2
  Demux1/1 -> Load DOBs/1
  Logical Operator1/1 -> Velocity Mode [true/false] x4/1
  [ResetSeaControl] -> Load Motion Disturbance Observer (Swing) Error-Proportional - 2nd order/1(reset)
  [ResetSeaControl] -> Desired Torque Derivative/2(Reset [1/0] x4)
  [DesiredSeaTorques] -> Compare SEA Signals/1(Desired)
  Selector11/1 -> [DesiredLateralTorques]
  Desired Torque [Nm] x6/1 -> Selector10/1, Selector11/1
  [LoadVelocities] -> Load Motion Disturbance Observer (Swing) Error-Proportional - 2nd order/4(velocities)
  [LoadPositions] -> Load Motion Disturbance Observer (Swing) Error-Proportional - 2nd order/3(positions)
  Selector5/1 -> [LoadVelocities]
  Selector1/1 -> [LoadPositions]
  [MeasuredSpringTorques] -> Load Motion Disturbance Observer (Swing) Error-Proportional - 2nd order/2(spring_torques)
  [MeasuredSpringTorques] -> Compare SEA Signals/2(Measured)
  Load Motion Disturbance Observer (Swing) Error-Proportional - 2nd order/1(d_hat_tp1) -> Unit Delay1/1
  Compare Velocities/2(RF) -> Desired vs Measured Motor Velocity/2
  Compare Velocities/1(RB) -> Desired vs Measured Motor Velocity/1
  Compare Velocities/3(LB) -> Desired vs Measured Motor Velocity/3
  Compare Velocities/4(LF) -> Desired vs Measured Motor Velocity/4
  Compare SEA Signals/4(LF) -> Desired vs Measured SEA Torques/4
  Compare SEA Signals/3(LB) -> Desired vs Measured SEA Torques/3
  Compare SEA Signals/2(RF) -> Desired vs Measured SEA Torques/2
  Compare SEA Signals/1(RB) -> Desired vs Measured SEA Torques/1
  Hip Motor Efficiency Compensation/1 -> Mux3/2, Sagittal and Lateral Motor Commands/2
  SEA Controller (Torque)/1(tau_cmd sagittal [Nm] x4) -> Mux3/1, Sagittal and Lateral Motor Commands/1
  Desired Torque Derivative/1(Derivative x4) -> SEA Controller (Torque)/6(dtau_des sagittal [Nm] x4)
  Mux3/1 -> Selector8/1
  [DesiredLateralTorques] -> Hip Motor Efficiency Compensation/1
  [DesiredSeaTorques] -> Desired Torque Derivative/1(Signal x4), SEA Controller (Torque)/5(tau_des sagittal [Nm] x4)
  [LoadPositions] -> SEA Controller (Torque)/1(phi_load [rad] x4)
  q/1 -> Selector3/1, Selector1/1
  Selector8/1 -> Torque Commands [Nm] x6/1
  SEA Controller (Torque)/2(tau_measured [Nm] x4) -> [MeasuredSpringTorques]
  [GearVelocities] -> SEA Controller (Torque)/4(dphi_gear [rad/s] x4)
  [StanceOrSwing] -> Logical Operator1/1
  Constant1/1 -> Stance or Swing1/2(Signal True x4)
